simulink model "ball_balancing_omni3_multibody_cascade_level_support"  (R2026a)
settings: Solver=ode15s  StopTime=ballbotParams.simulation.stopTime  MaxStep=ballbotParams.simulation.maxStep  RelTol=ballbotParams.simulation.relativeTolerance
PreLoadFcn:
  | ballbotParams = ballbotParameters; ballbotParams.controller.minimumContactConfidence = 0.10;
undefined symbols (not defined in the file): ballbotCascadeBalanceAllocate, ballbotEstimatorInitialState, ballbotEstimatorUpdate, ballbotImuFromJoint, ballbotPoseFromJoint, ballbotServoTorqueEnvelope, ballbotVelocityErrorBody, ballbotWheelRateFromDisplacement, X, Y, Z
libraries: sm_lib x29, nesl_utility x23
(part 1 of 3)
settings Model: Creator=cafdr  LastModifiedBy=cafdr
settings SimscapeCC: SimscapeLogType=none

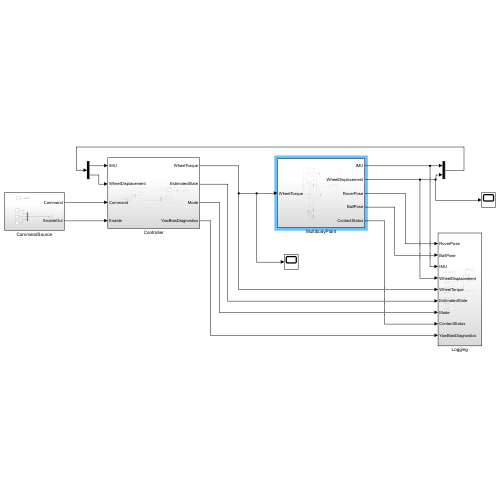
[thumbnail: Simulink's stored preview of the top-level diagram]
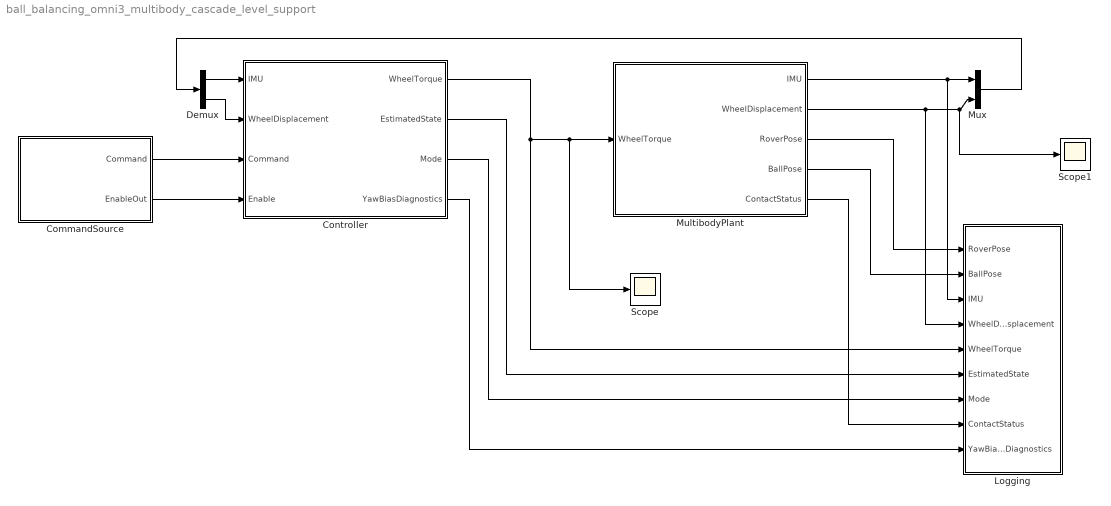
== system ball_balancing_omni3_multibody_cascade_level_support ==
  CommandSource : Subsystem
  Controller : Subsystem
  Demux : Demux  Outputs=2
  Logging : Subsystem
  MultibodyPlant : Subsystem
  Mux : Mux  Inputs=2
  Scope : Scope
      settings: ActiveDisplayYMinimum=-0.093711621357693731  ActiveDisplayYMaximum=0.065982668597649563
  Scope1 : Scope
      settings: ActiveDisplayYMinimum=-51.436545972709716  ActiveDisplayYMaximum=52.142033223021834
  wires:
  CommandSource/2(EnableOut) -> Controller/4(Enable)
  CommandSource/1(Command) -> Controller/3(Command)
  Mux/1 -> Demux/1
  Demux/1 -> Controller/1(IMU)
  Demux/2 -> Controller/2(WheelDisplacement)
  Controller/4(YawBiasDiagnostics) -> Logging/9(YawBiasDiagnostics)
  MultibodyPlant/2(WheelDisplacement) -> Scope1/1, Mux/2, Logging/4(WheelDisplacement)
  MultibodyPlant/1(IMU) -> Mux/1, Logging/3(IMU)
  Controller/1(WheelTorque) -> Logging/5(WheelTorque), Scope/1, MultibodyPlant/1(WheelTorque)
  MultibodyPlant/3(RoverPose) -> Logging/1(RoverPose)
  MultibodyPlant/4(BallPose) -> Logging/2(BallPose)
  Controller/2(EstimatedState) -> Logging/6(EstimatedState)
  Controller/3(Mode) -> Logging/7(Mode)
  MultibodyPlant/5(ContactStatus) -> Logging/8(ContactStatus)

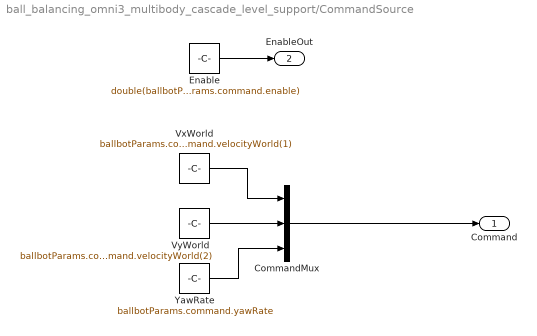
== system ball_balancing_omni3_multibody_cascade_level_support/CommandSource ==
  CommandMux : Mux  Inputs=3
  Enable : Constant  Value=double(ballbotParams.command.enable)  SampleTime=ballbotParams.controller.sampleTime
  VxWorld : Constant  Value=ballbotParams.command.velocityWorld(1)  SampleTime=ballbotParams.controller.sampleTime
  VyWorld : Constant  Value=ballbotParams.command.velocityWorld(2)  SampleTime=ballbotParams.controller.sampleTime
  YawRate : Constant  Value=ballbotParams.command.yawRate  SampleTime=ballbotParams.controller.sampleTime
  Command : Outport
  EnableOut : Outport  Port=2
  wires:
  Enable/1 -> EnableOut/1
  YawRate/1 -> CommandMux/3
  VxWorld/1 -> CommandMux/1
  VyWorld/1 -> CommandMux/2
  CommandMux/1 -> Command/1

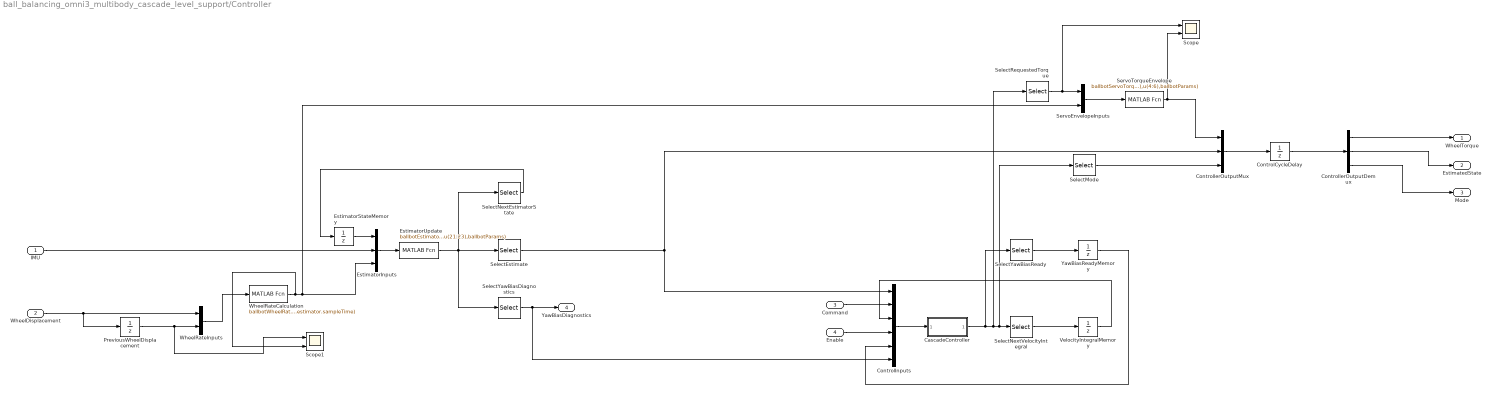
== system ball_balancing_omni3_multibody_cascade_level_support/Controller ==
  IMU : Inport  PortDimensions=6
  WheelDisplacement : Inport  Port=2  PortDimensions=3
  Command : Inport  Port=3
  Enable : Inport  Port=4
  CascadeController : Subsystem
  ControlCycleDelay : UnitDelay  InitialCondition=zeros(18,1)  SampleTime=ballbotParams.controller.sampleTime
  ControlInputs : Mux  Inputs=6
  ControllerOutputDemux : Demux  Outputs=[3 14 1]
  ControllerOutputMux : Mux  Inputs=3
  EstimatorInputs : Mux  Inputs=3
  EstimatorStateMemory : UnitDelay  InitialCondition=ballbotEstimatorInitialState  SampleTime=ballbotParams.controller.sampleTime
  EstimatorUpdate : MATLABFcn  MATLABFcn=ballbotEstimatorUpdate(u(1:14),u(15:20),u(21:23),ballbotParams)  OutputDimensions=31  SampleTime=ballbotParams.controller.sampleTime
  PreviousWheelDisplacement : UnitDelay  InitialCondition=zeros(3,1)  SampleTime=ballbotParams.controller.sampleTime
  Scope : Scope  NumInputPorts=2
      settings: ActiveDisplayYMinimum=-1  ActiveDisplayYMaximum=1  DataLoggingVariableName=ScopeData2
  Scope1 : Scope  NumInputPorts=2
      settings: ActiveDisplayYMinimum=-29.766814569729064  ActiveDisplayYMaximum=10.416225049193823  DataLoggingVariableName=ScopeData3
  SelectEstimate : Selector  InputPortWidth=31  IndexOptions=Index vector (dialog)  Indices=15:28  OutputSizes=1
  SelectMode : Selector  InputPortWidth=7  IndexOptions=Index vector (dialog)  Indices=6  OutputSizes=1
  SelectNextEstimatorState : Selector  InputPortWidth=31  IndexOptions=Index vector (dialog)  Indices=1:14  OutputSizes=1
  SelectNextVelocityIntegral : Selector  InputPortWidth=7  IndexOptions=Index vector (dialog)  Indices=4:5  OutputSizes=1
  SelectRequestedTorque : Selector  InputPortWidth=7  IndexOptions=Index vector (dialog)  Indices=1:3  OutputSizes=1
  SelectYawBiasDiagnostics : Selector  InputPortWidth=31  IndexOptions=Index vector (dialog)  Indices=29:31  OutputSizes=1
  SelectYawBiasReady : Selector  InputPortWidth=7  IndexOptions=Index vector (dialog)  Indices=7  OutputSizes=1
  ServoEnvelopeInputs : Mux  Inputs=2
  ServoTorqueEnvelope : MATLABFcn  MATLABFcn=ballbotServoTorqueEnvelope(u(1:3),u(4:6),ballbotParams)  OutputDimensions=3  SampleTime=ballbotParams.controller.sampleTime
  VelocityIntegralMemory : UnitDelay  InitialCondition=zeros(2,1)  SampleTime=ballbotParams.controller.sampleTime
  WheelRateCalculation : MATLABFcn  MATLABFcn=ballbotWheelRateFromDisplacement(u(1:3),u(4:6),ballbotParams.estimator.sampleTime)  OutputDimensions=3  SampleTime=ballbotParams.controller.sampleTime
  WheelRateInputs : Mux  Inputs=2
  YawBiasReadyMemory : UnitDelay  SampleTime=ballbotParams.controller.sampleTime
  WheelTorque : Outport
  EstimatedState : Outport  Port=2
  Mode : Outport  Port=3
  YawBiasDiagnostics : Outport  Port=4
  wires:
  ServoEnvelopeInputs/1 -> ServoTorqueEnvelope/1
  SelectRequestedTorque/1 -> Scope/1, ServoEnvelopeInputs/1
  SelectNextVelocityIntegral/1 -> VelocityIntegralMemory/1
  SelectNextEstimatorState/1 -> EstimatorStateMemory/1
  EstimatorInputs/1 -> EstimatorUpdate/1
  WheelRateCalculation/1 -> Scope1/2, EstimatorInputs/3, ServoEnvelopeInputs/2
  IMU/1 -> EstimatorInputs/2
  EstimatorStateMemory/1 -> EstimatorInputs/1
  WheelRateInputs/1 -> WheelRateCalculation/1
  PreviousWheelDisplacement/1 -> Scope1/1, WheelRateInputs/2
  WheelDisplacement/1 -> PreviousWheelDisplacement/1, WheelRateInputs/1
  ControlCycleDelay/1 -> ControllerOutputDemux/1
  ControllerOutputDemux/3 -> Mode/1
  ControllerOutputDemux/1 -> WheelTorque/1
  ControllerOutputDemux/2 -> EstimatedState/1
  ServoTorqueEnvelope/1 -> Scope/2, ControllerOutputMux/1
  SelectMode/1 -> ControllerOutputMux/3
  ControllerOutputMux/1 -> ControlCycleDelay/1
  EstimatorUpdate/1 -> SelectNextEstimatorState/1, SelectEstimate/1, SelectYawBiasDiagnostics/1
  YawBiasReadyMemory/1 -> ControlInputs/5
  SelectYawBiasReady/1 -> YawBiasReadyMemory/1
  SelectYawBiasDiagnostics/1 -> YawBiasDiagnostics/1, ControlInputs/6
  SelectEstimate/1 -> ControllerOutputMux/2, ControlInputs/1
  Command/1 -> ControlInputs/2
  VelocityIntegralMemory/1 -> ControlInputs/3
  Enable/1 -> ControlInputs/4
  ControlInputs/1 -> CascadeController/1(ControlVector)
  CascadeController/1(ControllerOutput) -> SelectNextVelocityIntegral/1, SelectMode/1, SelectRequestedTorque/1, SelectYawBiasReady/1

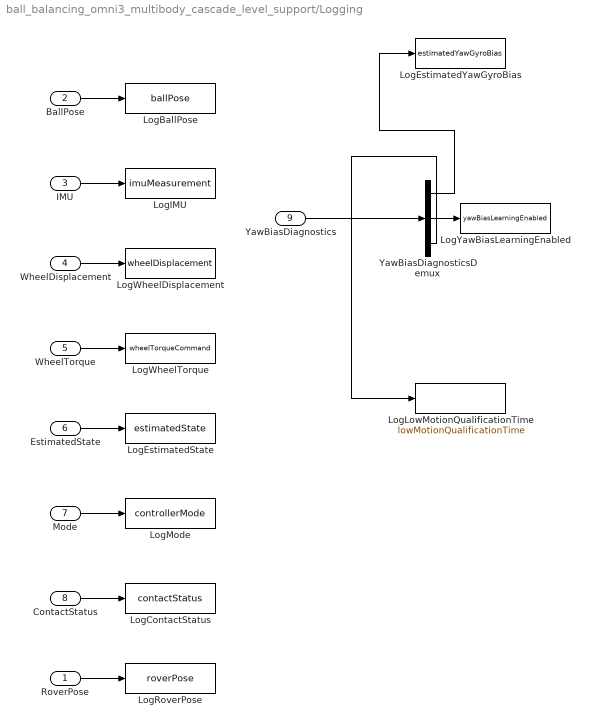
== system ball_balancing_omni3_multibody_cascade_level_support/Logging ==
  RoverPose : Inport
  BallPose : Inport  Port=2
  IMU : Inport  Port=3
  WheelDisplacement : Inport  Port=4
  WheelTorque : Inport  Port=5
  EstimatedState : Inport  Port=6
  Mode : Inport  Port=7
  ContactStatus : Inport  Port=8
  YawBiasDiagnostics : Inport  Port=9
  LogBallPose : ToWorkspace  VariableName=ballPose  SaveFormat=Timeseries  SampleTime=-1
  LogContactStatus : ToWorkspace  VariableName=contactStatus  SaveFormat=Timeseries  SampleTime=-1
  LogEstimatedState : ToWorkspace  VariableName=estimatedState  SaveFormat=Timeseries  SampleTime=-1
  LogEstimatedYawGyroBias : ToWorkspace  VariableName=estimatedYawGyroBias  SaveFormat=Timeseries  SampleTime=-1
  LogIMU : ToWorkspace  VariableName=imuMeasurement  SaveFormat=Timeseries  SampleTime=-1
  LogLowMotionQualificationTime : ToWorkspace  VariableName=lowMotionQualificationTime  SaveFormat=Timeseries  SampleTime=-1
  LogMode : ToWorkspace  VariableName=controllerMode  SaveFormat=Timeseries  SampleTime=-1
  LogRoverPose : ToWorkspace  VariableName=roverPose  SaveFormat=Timeseries  SampleTime=-1
  LogWheelDisplacement : ToWorkspace  VariableName=wheelDisplacement  SaveFormat=Timeseries  SampleTime=-1
  LogWheelTorque : ToWorkspace  VariableName=wheelTorqueCommand  SaveFormat=Timeseries  SampleTime=-1
  LogYawBiasLearningEnabled : ToWorkspace  VariableName=yawBiasLearningEnabled  SaveFormat=Timeseries  SampleTime=-1
  YawBiasDiagnosticsDemux : Demux  Outputs=3
  wires:
  ContactStatus/1 -> LogContactStatus/1
  Mode/1 -> LogMode/1
  EstimatedState/1 -> LogEstimatedState/1
  WheelTorque/1 -> LogWheelTorque/1
  WheelDisplacement/1 -> LogWheelDisplacement/1
  IMU/1 -> LogIMU/1
  BallPose/1 -> LogBallPose/1
  RoverPose/1 -> LogRoverPose/1
  YawBiasDiagnosticsDemux/3 -> LogLowMotionQualificationTime/1
  YawBiasDiagnosticsDemux/2 -> LogYawBiasLearningEnabled/1
  YawBiasDiagnosticsDemux/1 -> LogEstimatedYawGyroBias/1
  YawBiasDiagnostics/1 -> YawBiasDiagnosticsDemux/1
